simulink model "simulink_sui"  (R2020a)
settings: Solver=VariableStepAuto  StartTime=0.0  StopTime=25.0  RelTol=1e-3
values from neighbouring files (symbols this model uses):
  a = -1/T    (= -0.2)    [Plotting.m]    (also in Task33_advancedexpressions.m = 1; brackets.m = [2+2]*2; checkifprime.m = 'The given number is not a prime number'; dheg.m = 1)
  x0 = 1    [Plotting.m]
settings Model: Creator=Dhanush Wagle  LastModifiedBy=Dhanush Wagle

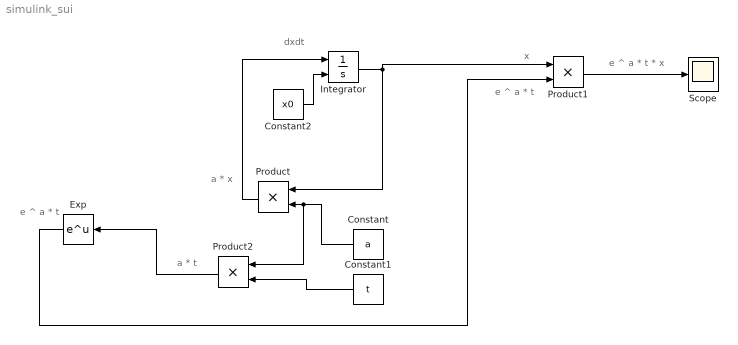
== system simulink_sui ==
  note: e ^ a * t * x
  note: e ^ a * t
  note: a * t
  note: a * x
  note: dxdt
  note: x
  note: e ^ a * t
  Constant : Constant  Value=a
  Constant1 : Constant  Value=t
  Constant2 : Constant  Value=x0
  Exp : Math  SaturateOnIntegerOverflow=on
  Integrator : Integrator  InitialConditionSource=external
  Product : Product
  Product1 : Product
  Product2 : Product
  Scope : Scope
  wires:
  Integrator/1 -> Product1/1, Product/1
  Constant/1 -> Product2/1, Product/2
  Product/1 -> Integrator/1
  Product2/1 -> Exp/1
  Constant1/1 -> Product2/2
  Exp/1 -> Product1/2
  Product1/1 -> Scope/1
  Constant2/1 -> Integrator/2
